simulink model "Simulink_Block_Diagrams"  (R2025b)
settings: Solver=ode15s  StartTime=0.0  StopTime=0.01  RelTol=1e-3
values from neighbouring files (symbols this model uses):
  iL = min(max(iL, 0), 20)    [ece141-matlab.m]
  Kd = 0.00025    [a.mat]    (also in ece141-matlab.m)
  vdc0 = 80    [a.mat]    (also in ece141-matlab.m)
  vs0 = 80    [a.mat]    (also in ece141-matlab.m)
libraries: slpidlib x1
settings Model: Creator=wesle  LastModifiedBy=wesle

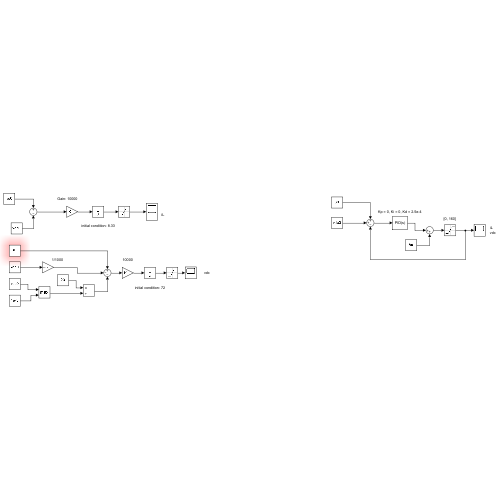
[thumbnail: Simulink's stored preview of the top-level diagram]
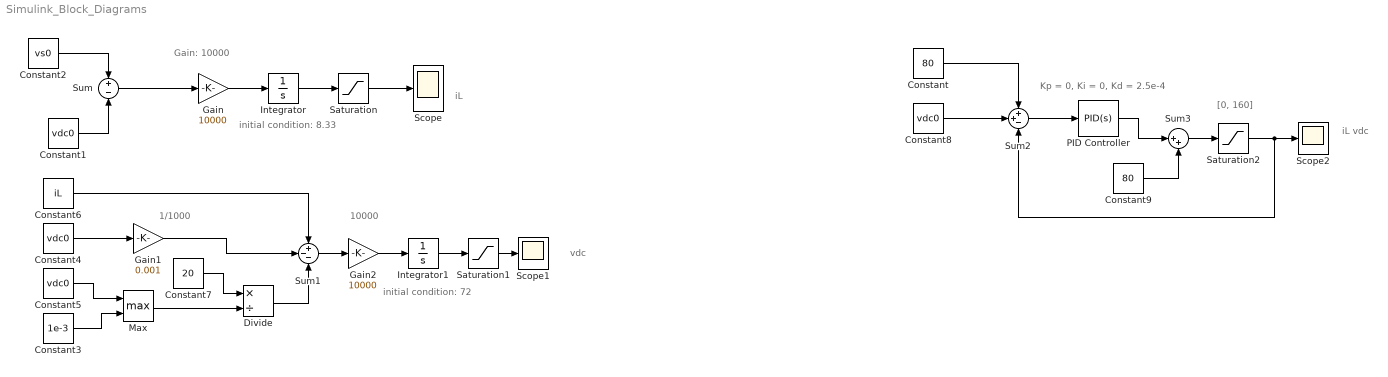
== system Simulink_Block_Diagrams ==
  note: iL
      | vdc
  note: [0, 160]
  note: Kp = 0, Ki = 0, Kd = 2.5e-4
  note: initial condition: 72
  note: vdc
  note: 10000
  note: 1/1000
  note: iL
  note: Gain: 10000
  note: initial condition: 8.33
  Constant : Constant  Value=80
  Constant{1,4..5,8} (4 alike) : Constant  Value=vdc0
  Constant2 : Constant  Value=vs0
  Constant3 : Constant  Value=1e-3
  Constant6 : Constant  Value=iL
  Constant7 : Constant  Value=20
  Constant9 : Constant  Value=80
  Divide : Product  Inputs=*/
  Gain : Gain  Gain=10000
  Gain1 : Gain  Gain=0.001
  Gain2 : Gain  Gain=10000
  Integrator : Integrator  InitialCondition=8.33
  Integrator1 : Integrator  InitialCondition=72
  Max : MinMax  Function=max  Inputs=2
  PID Controller : slpidlib/PID Controller  Controller=PID  Form=Parallel  TimeDomain=Continuous-time  UseExternalTs=off  SampleTime=-1  IntegratorMethod=Forward Euler  FilterMethod=Forward Euler  ControllerParametersSource=internal  P=0  I=0  UseKiTs=off  D=Kd  UseExternalDerivativeSource=off  N=100  UseFilter=on  TunerSelectOption=Transfer Function Based (PID Tuner App)  InitialConditionSource=internal  InitialConditionForIntegrator=0  InitialConditionForFilter=0  DifferentiatorICPrevScaledInput=0  ExternalReset=none  TrackingMode=off  Kt=1  LimitOutput=off  SatLimitsSource=internal  UpperSaturationLimit=inf  LowerSaturationLimit=-inf  LinearizeAsGain=on  AntiWindupMode=none  Kb=1  LimitIntegrator=off  UpperIntegratorSaturationLimit=inf  LowerIntegratorSaturationLimit=-inf  POutMin=[]  POutMax=[]  IOutMin=[]  IOutMax=[]  DOutMin=[]  DOutMax=[]  NOutMin=[]  NOutMax=[]  SumOutMin=[]  SumOutMax=[]  SaturationOutMin=[]  SaturationOutMax=[]  PParamMin=[]  PParamMax=[]  IParamMin=[]  IParamMax=[]  DParamMin=[]  DParamMax=[]  NParamMin=[]  NParamMax=[]  KbParamMin=[]  KbParamMax=[]  KtParamMin=[]  KtParamMax=[]  KbOutMin=[]  KbOutMax=[]  KtOutMin=[]  KtOutMax=[]  IntegratorOutMin=[]  IntegratorOutMax=[]  FilterOutMin=[]  FilterOutMax=[]  SumI1OutMin=[]  SumI1OutMax=[]  SumI2OutMin=[]  SumI2OutMax=[]  SumI3OutMin=[]  SumI3OutMax=[]  SumI4OutMin=[]  SumI4OutMax=[]  SumDOutMin=[]  SumDOutMax=[]  DifferentiatorOutMin=[]  DifferentiatorOutMax=[]  FilterDiffOutCoefMin=[]  FilterDiffOutCoefMax=[]  ReciprocalOutMin=[]  ReciprocalOutMax=[]  SumDenOutMin=[]  SumDenOutMax=[]  SumNumOutMin=[]  SumNumOutMax=[]  DivideOutMin=[]  DivideOutMax=[]  UdiffTsProdOutMin=[]  UdiffTsProdOutMax=[]  NTsProdOutMin=[]  NTsProdOutMax=[]  UintegralTsProdOutMin=[]  UintegralTsProdOutMax=[]  UngainTsProdOutMin=[]  UngainTsProdOutMax=[]  ClampingZeroOutDataTypeStr=Inherit: Inherit via back propagation  ClampingZeroOutMin=[]  ClampingZeroOutMax=[]  FilterDenConstantOutDataTypeStr=Inherit: Inherit via back propagation  FilterDenConstantOutMin=[]  FilterDenConstantOutMax=[]  PCopyOutDataTypeStr=Inherit: Inherit via back propagation  PCopyOutMin=[]  PCopyOutMax=[]  NCopyOutDataTypeStr=Inherit: Inherit via back propagation  NCopyOutMin=[]  NCopyOutMax=[]  IntegratorContinuousStateAttributes=''  IntegratorStateMustResolveToSignalObject=off  IntegratorRTWStateStorageClass=Auto  FilterContinuousStateAttributes=''  FilterStateMustResolveToSignalObject=off  FilterRTWStateStorageClass=Auto  ParallelPVariant=InternalParameters  IdealPVariant=Disabled  IVariant=InternalParameters  DVariant=InternalParameters  IntegratorVariant=Continuous  SatVariant=Disabled  AWVariant=Passthrough  PCopyVariant=Disabled  TRVariant=Disabled  FdbkBlocksVariant=Forward  IdealPFdbkVariant=Disabled  SatFdbkVariant=Disabled  DerivativeFilterVariant=ContFilter  NVariant=InternalParameters  NCopyVariant=Disabled  FilterICVariant=InternalICsFilter  IntegratorICVariant=InternalICs  ExternalResetVariant=Disabled  TRSumVariant=Passthrough  SumFdbkVariant=Disabled  SumVariant=Sum_PID  TsampFilterVariant=InternalTs  TsampNgainVariant=Passthrough  TsampIntegralVariant=Disabled_SignalSpec  ExternalSaturationOutDataTypeStr=Inherit: Same as second input  DerivativeSourceVariant=ErrorSignal  PreIntVariant=InternalPreInt
  Saturation : Saturate  UpperLimit=20  LowerLimit=0
  Saturation1 : Saturate  UpperLimit=200  LowerLimit=0
  Saturation2 : Saturate  UpperLimit=160  LowerLimit=0
  Scope : Scope
  Scope1 : Scope
  Scope2 : Scope
      settings: DataLoggingVariableName=ScopeData2
  Sum : Sum  Inputs=+-
  Sum1 : Sum  Inputs=+--
  Sum2 : Sum  Inputs=++-
  Sum3 : Sum  Inputs=|++
  wires:
  Constant2/1 -> Sum/1
  Constant1/1 -> Sum/2
  Sum/1 -> Gain/1
  Gain/1 -> Integrator/1
  Constant6/1 -> Sum1/1
  Constant4/1 -> Gain1/1
  Gain1/1 -> Sum1/2
  Constant5/1 -> Max/1
  Constant3/1 -> Max/2
  Constant7/1 -> Divide/1
  Max/1 -> Divide/2
  Divide/1 -> Sum1/3
  Sum1/1 -> Gain2/1
  Saturation/1 -> Scope/1
  Integrator/1 -> Saturation/1
  Gain2/1 -> Integrator1/1
  Saturation1/1 -> Scope1/1
  Integrator1/1 -> Saturation1/1
  Constant/1 -> Sum2/1
  Constant8/1 -> Sum2/2
  Sum2/1 -> PID Controller/1
  PID Controller/1 -> Sum3/1
  Constant9/1 -> Sum3/2
  Sum3/1 -> Saturation2/1
  Saturation2/1 -> Sum2/3, Scope2/1
